simulink model "simu_test"  (R2016a)
settings: Solver=VariableStepAuto  StartTime=0.0  StopTime=10.0  RelTol=1e-3
settings Model: Creator=manuel  LastModifiedBy=manuel
settings GRTTargetCC: GeneratePreprocessorConditionals=Use local settings

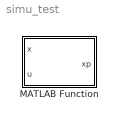
== system simu_test ==
  MATLAB Function : MATLAB Function  TreatAsAtomicUnit=on

== matlab function simu_test/MATLAB Function ==
  data: x input; u input; xp output
function xp = fcn(x,u)
%#codegen
[A,B] = return_values();
xp = A*x + B*u;
